simulink subsystem "Autonomous_sub"  (R2023b)
settings: Solver=VariableStepAuto  StartTime=0.0  StopTime=10.0  RelTol=1e-3
undefined symbols (not defined in the file): Auto_Signal_two
libraries: simulink x2
settings Model: Creator=ander  LastModifiedBy=ander

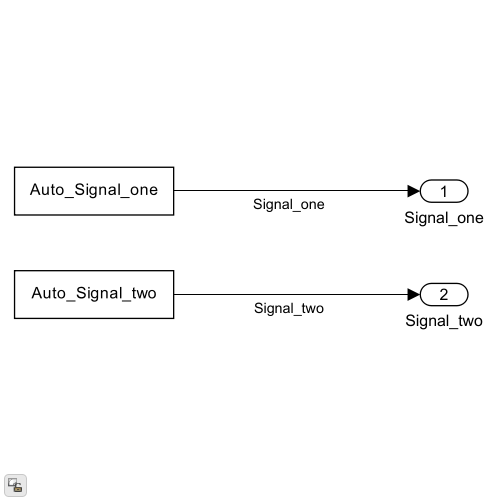
[thumbnail: Simulink's stored preview of the top-level diagram]
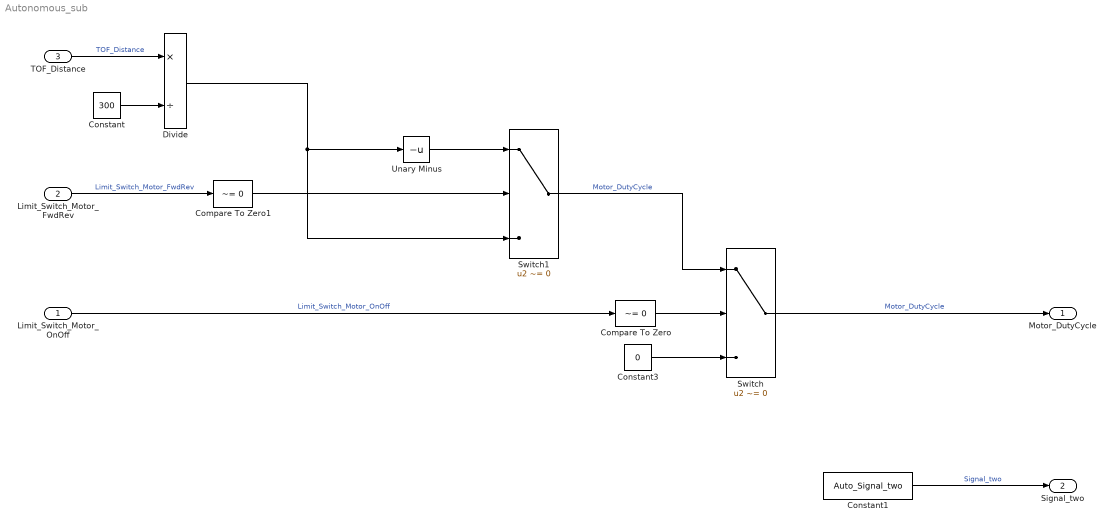
== system Autonomous_sub ==
  Limit_Switch_Motor_OnOff : Inport
  Limit_Switch_Motor_FwdRev : Inport  Port=2
  TOF_Distance : Inport  Port=3
  Compare To Zero : simulink/Logic and Bit Operations/Compare To Zero  relop=~=  OutDataTypeStr=boolean
  Compare To Zero1 : simulink/Logic and Bit Operations/Compare To Zero  relop=~=  OutDataTypeStr=boolean
  Constant : Constant  Value=300
  Constant1 : Constant  Value=Auto_Signal_two
  Constant3 : Constant  Value=0
  Divide : Product  Inputs=*/
  Switch : Switch  Criteria=u2 ~= 0  SaturateOnIntegerOverflow=off  InputSameDT=off
  Switch1 : Switch  Criteria=u2 ~= 0  SaturateOnIntegerOverflow=off  InputSameDT=off
  Unary Minus : UnaryMinus
  Motor_DutyCycle : Outport
  Signal_two : Outport  Port=2
  wires:
  Constant1/1 -> Signal_two/1  "Signal_two"
  Switch/1 -> Motor_DutyCycle/1  "Motor_DutyCycle"
  Compare To Zero/1 -> Switch/2
  Limit_Switch_Motor_OnOff/1 -> Compare To Zero/1  "Limit_Switch_Motor_OnOff"
  Constant3/1 -> Switch/3
  Switch1/1 -> Switch/1  "Motor_DutyCycle"
  Limit_Switch_Motor_FwdRev/1 -> Compare To Zero1/1  "Limit_Switch_Motor_FwdRev"
  Compare To Zero1/1 -> Switch1/2
  TOF_Distance/1 -> Divide/1  "TOF_Distance"
  Constant/1 -> Divide/2
  Divide/1 -> Unary Minus/1, Switch1/3
  Unary Minus/1 -> Switch1/1
